simulink model "power_hvdc"  (Simulink 6.0)
settings: Solver=FixedStepDiscrete  SolverMode=SingleTasking  StartTime=0.0  StopTime=0.8  RelTol=1e-4
undefined symbols (not defined in the file or in its folder): D1, Delta
libraries: powerlib x28, powerlib_extras x7
settings Model: Creator=patrice  LastModifiedBy=batserve  ExtModeTrigMode=oneshot  ExtModeArmWhenConnect=off  ExtModeAutoUpdateStatusClock=off
settings DataIOCC: LimitDataPoints=off  SaveOutput=off  TimeSaveName=t  SignalLoggingName=sigsOut
settings OptimizationCC: BlockReduction=off  BooleanDataType=off
settings DebuggingCC: CheckExecutionContextPreStartOutputMsg=on  CheckExecutionContextRuntimeOutputMsg=on  SolverPrmCheckMsg=none
settings HardwareCC: TargetUnknown=on
settings RTWCC: TemplateMakefile=grt_unix.tmf

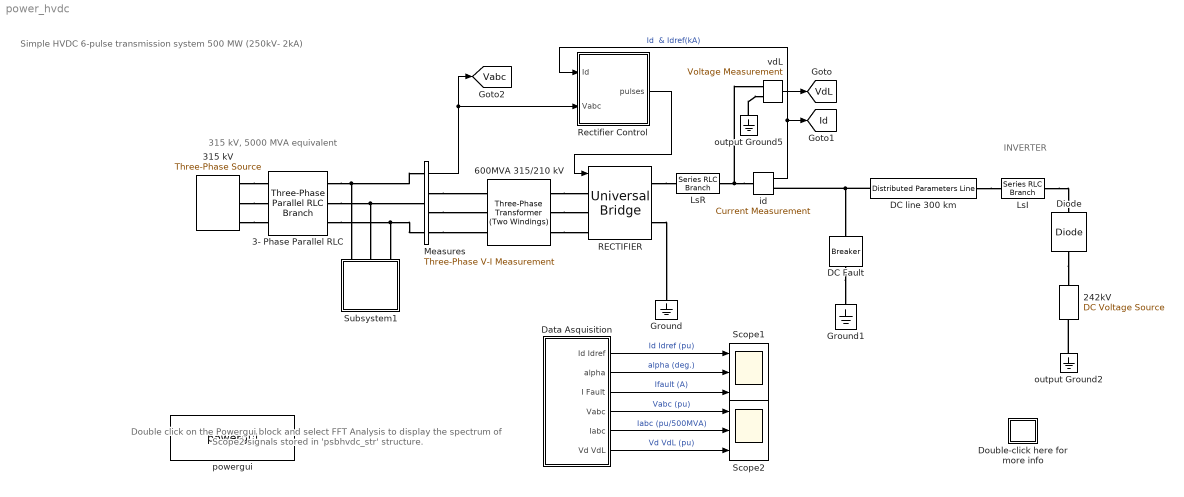
== system power_hvdc ==
  note: INVERTER
  note: Simple HVDC 6-pulse transmission system
      | 500 MW (250kV- 2kA)
  note: 315 kV, 5000 MVA equivalent
  note: Double click on the Powergui block
      | and select  FFT Analysis to display
      | the spectrum of Scope2  signals
      | stored in 'psbhvdc_str' structure.
  242kV : powerlib/Electrical Sources/DC Voltage Source  Description=source block  Orientation=up  Amplitude=242000  Measurements=None
      settings: AttributesFormatString=\n
  3- Phase Parallel RLC : powerlib/Elements/Three-Phase Parallel RLC Branch  PhysicalDomain=powersysdomain  SubClassName=unknown  LeftPortType=p1  RightPortType=p1  LConnTagsString=A|B|C  RConnTagsString=A|B|C  Resistance=12.41  Inductance=23.264e-3  Capacitance=0  Measurements=None
  315 kV : powerlib/Electrical Sources/Three-Phase Source  Voltage=315e3  PhaseAngle=0  Frequency=60  InternalConnection=Yg  SpecifyImpedance=off  Resistance=0  Inductance=46.671e-3  ShortCircuitLevel=0  BaseVoltage=0  XRratio=0
  600MVA 315/210 kV : powerlib/Elements/Three-Phase Transformer (Two Windings)  NominalPower=[ 600e6 60 ]  Winding1Connection=Yg  Winding1="[ 315e3*0.97 0.0015  0.0 ]"  Winding2Connection=Delta (D1)  Winding2=[ 210e3 0.0015 0.12]  SetSaturation=off  Rm=500  Lm=500  Saturation="[ 0,0  ;  0.005,1.2  ;  1.0,1.4 ]"  Hysteresis=off  DataFile='hysteresis'  SetInitialFlux=off  InitialFluxes=[ 0.8 , -0.8 , 0.7 ]  Measurements=None  TransfoNumber=0
  DC Fault : powerlib/Elements/Breaker  Orientation=down  BreakerResistance=0.1  InitialState=0  SnubberResistance=inf  SnubberCapacitance=0  SwitchingTimes=[ 0.5 0.51 ]  External=off  Measurements=Branch current
      settings: AttributesFormatString=\n
  DC line 300 km : powerlib/Elements/Distributed Parameters Line  Phases=1  Frequency=60  Resistance=0.015  Inductance=0.792e-3  Capacitance=14.4e-9  Length=300  x1=[0 0 0 0; 0.0001244 0 0 0; 0.0002488 0 0 0; 0.0003733 0 0 0; 0.0004977 0 0 0; 0.0006221 0 0 0]  x2=[0 0 0 0; 0.0001244 0 0 0; 0.0002488 0 0 0; 0.0003733 0 0 0; 0.0004977 0 0 0; 0.0006221 0 0 0]  x3=[0 0 0 0; 0.0001244 0 0 0; 0.0002488 0 0 0; 0.0003733 0 0 0; 0.0004977 0 0 0; 0.0006221 0 0 0]  x4=[0 0 0 0; 0.0001244 0 0 0; 0.0002488 0 0 0; 0.0003733 0 0 0; 0.0004977 0 0 0; 0.0006221 0 0 0]  x5=0  Measurements=None
      settings: AttributesFormatString=\n
  Data Asquisition : Subsystem
  Diode : powerlib/Power Electronics/Diode  Orientation=down  Ron=0.01  Lon=0  Vf=0.8  IC=0  Rs=1000  Cs=0.05e-6  Measurements=off
  Double-click here for more info : Subsystem
      mask Display: disp('?')
  Ground : powerlib/Elements/Ground  Orientation=down  PhysicalDomain=powersysdomain  SubClassName=unknown  LeftPortType=p1  RightPortType=p1  LConnTagsString=a
  Ground1 : powerlib/Elements/Ground  Orientation=down  PhysicalDomain=powersysdomain  SubClassName=unknown  LeftPortType=p1  RightPortType=p1  LConnTagsString=a
  LsI : powerlib/Elements/Series RLC Branch  PhysicalDomain=powersysdomain  SubClassName=unknown  LeftPortType=p1  RightPortType=p1  LConnTagsString=__new0  RConnTagsString=__new0  Resistance=.5  Inductance=.5  Capacitance=inf  Measurements=None
  "LsR " : powerlib/Elements/Series RLC Branch  PhysicalDomain=powersysdomain  SubClassName=unknown  LeftPortType=p1  RightPortType=p1  LConnTagsString=__new0  RConnTagsString=__new0  Resistance=.5  Inductance=.5  Capacitance=inf  Measurements=None
  Measures : powerlib/Measurements/Three-Phase V-I Measurement  VoltageMeasurement=phase-to-ground  SetLabelV=off  LabelV=V1  Vpu=on  Vbase=315e3  CurrentMeasurement=yes  SetLabelI=on  LabelI=Iabc  Ipu=on  Pbase=500e6  OutputType=Magnitude  PhasorSimulation=off  PSBequivalent=0
  RECTIFIER : powerlib/Power Electronics/Universal Bridge  Arms=3  SnubberResistance=2000  SnubberCapacitance=50e-9  Device=Thyristors  Ron=1e-3  Lon=0  ForwardVoltages="[  0.8  0.8  ]"  ForwardVoltage=0  GTOparameters=[ 10e-6 , 20e-6 ]  IGBTparameters=[ 1e-6 , 2e-6 ]  Measurements=UAB UBC UCA UDC voltages
  Rectifier Control : Subsystem
  Scope1 : Scope  NumInputPorts=3
      settings: TimeRange=0.8  YMin=-0.25~0~-500  YMax=2~170~6000  DataFormat=Array
  Scope2 : Scope  NumInputPorts=3
      settings: TimeRange=0.8  YMin=-1.5~-3~-1.5  YMax=1.5~3~2  SaveName=psbhvdc_str
  Subsystem1 : Subsystem  Orientation=down
      mask Display: disp('AC filters \n(320 Mvar)')
  id : powerlib/Measurements/Current Measurement  Tag=PoWeRsYsTeMmEaSuReMeNt  PhasorSimulation=off  OutputType=Complex  PSBequivalent=0
  output Ground2 : powerlib/Elements/Ground  Orientation=down  PhysicalDomain=powersysdomain  SubClassName=unknown  LeftPortType=p1  RightPortType=p1  LConnTagsString=a
  output Ground5 : powerlib/Elements/Ground  Orientation=down  PhysicalDomain=powersysdomain  SubClassName=unknown  LeftPortType=p1  RightPortType=p1  LConnTagsString=a
  powergui : powerlib/powergui  Priority=2  Frange=[0:2:500]  Ylog=off  Xlog=off  save=off  variable=ZData  structure=psbhvdc_str  ZoomFFT=on  StartTime=0.8-2/60  cycles=2  DisplayStyle=off  fundamental=60  FreqAxis=on  MaxFrequency=2000  frequencyindice=1  frequencyindicesteady=1  RmsSteady=1  display=off  Ts=1/360/64  methode=off  frequency=60  echomessages=off
  vdL : powerlib/Measurements/Voltage Measurement  Tag=PoWeRsYsTeMmEaSuReMeNt  PhasorSimulation=off  OutputType=Complex  PSBequivalent=0
  tag scope: Id=global, Vabc=global, VdL=global
  wires:
  Data Asquisition/6(Vd VdL) -> Scope2/3  "Vd VdL (pu)"
  Data Asquisition/1("Id Idref ") -> Scope1/1  "Id Idref (pu)"
  Data Asquisition/3(I Fault) -> Scope1/3  "Ifault (A)"
  Data Asquisition/2(alpha) -> Scope1/2  "alpha (deg.)"
  Data Asquisition/4(Vabc) -> Scope2/1  "Vabc (pu)"
  Data Asquisition/5(Iabc) -> Scope2/2  "Iabc (pu/500MVA)"
  Rectifier Control/1(pulses) -> RECTIFIER/1
  id/1 -> Rectifier Control/1(Id), [Id]  "Id  & Idref(kA)"
  Measures/1 -> [Vabc], Rectifier Control/2(Vabc)
  vdL/1 -> [VdL]
  connections:
  RECTIFIER/RConn1 -- "LsR "/LConn1
  RECTIFIER/RConn2 -- Ground/LConn1
  600MVA 315/210 kV/RConn1 -- RECTIFIER/LConn1
  600MVA 315/210 kV/RConn2 -- RECTIFIER/LConn2
  600MVA 315/210 kV/RConn3 -- RECTIFIER/LConn3
  Measures/RConn1 -- 600MVA 315/210 kV/LConn1
  Measures/RConn2 -- 600MVA 315/210 kV/LConn2
  Measures/RConn3 -- 600MVA 315/210 kV/LConn3
  DC line 300 km/RConn1 -- LsI/LConn1
  DC line 300 km/LConn1 -- id/RConn1 -- DC Fault/LConn1
  "LsR "/RConn1 -- id/LConn1 -- vdL/LConn1
  output Ground5/LConn1 -- vdL/LConn2
  DC Fault/RConn1 -- Ground1/LConn1
  output Ground2/LConn1 -- 242kV/LConn1
  LsI/RConn1 -- Diode/LConn1
  315 kV/RConn1 -- 3- Phase Parallel RLC/LConn1
  315 kV/RConn2 -- 3- Phase Parallel RLC/LConn2
  315 kV/RConn3 -- 3- Phase Parallel RLC/LConn3
  Diode/RConn1 -- 242kV/RConn1
  3- Phase Parallel RLC/RConn2 -- Measures/LConn2 -- Subsystem1/LConn2
  3- Phase Parallel RLC/RConn1 -- Measures/LConn1 -- Subsystem1/LConn1
  3- Phase Parallel RLC/RConn3 -- Measures/LConn3 -- Subsystem1/LConn3

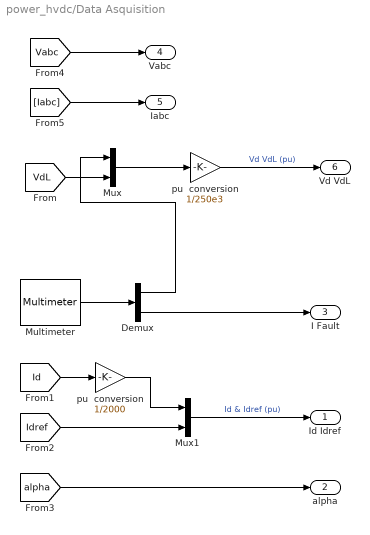
== system power_hvdc/Data Asquisition ==
  Demux : Demux  Outputs=2
  Multimeter : powerlib/Measurements/Multimeter  Tag=PoWeRsYsTeMmEaSuReMeNt  PhasorSimulation=off  OutputType=Magnitude  sel=[4 5]  L=5  Gain=[1 1]  yselected={'Udc: RECTIFIER','Ib: DC Fault'};  PSBOutputType=1  PSBequivalent=0  AxesSetting=[0,0.1,-100,100]  Display=0  SavedBlockNames={}
      settings: AttributesFormatString=\n
  Mux : Mux  Inputs=2
  Mux1 : Mux  Inputs=2
  pu  conversion : Gain  Gain=1/2000  SaturateOnIntegerOverflow=on
  "pu  conversion " : Gain  Gain=1/250e3  SaturateOnIntegerOverflow=on
  "Id Idref " : Outport
  alpha : Outport  Port=2
  I Fault : Outport  Port=3
  Vabc : Outport  Port=4
  Iabc : Outport  Port=5
  Vd VdL : Outport  Port=6
  wires:
  Mux/1 -> "pu  conversion "/1
  [VdL] -> Mux/2
  [Id] -> pu  conversion/1
  Mux1/1 -> "Id Idref "/1  "Id & Idref (pu)"
  [Idref] -> Mux1/2
  Demux/2 -> I Fault/1
  Demux/1 -> Mux/1
  [alpha] -> alpha/1
  [Vabc] -> Vabc/1
  [Iabc] -> Iabc/1
  "pu  conversion "/1 -> Vd VdL/1  "Vd VdL (pu)"
  pu  conversion/1 -> Mux1/1
  Multimeter/1 -> Demux/1

== system power_hvdc/Double-click here for more info ==
  note: Note: In oder to appreciate the speed improvemnt obtained with discretisation, you may try continuous simulation mode after completing this demo.
      |          The discrete system is approximately 6 times faster.
  note: Notice that the system is discretized (sample time 1/360/64 = 43.4 us). Setting, the sample time in to zero, will change to continuous integration for the power system .
  note: Frequency analysis of AC and DC voltages and currents
  note: In order to alllow further signal processing, signals displayed on Scope2 have been saved in a variable named 'psbvdc_str' ( structure with time').
      | These signals are : AC voltages (input 1) , AC currents (input 2) and DC voltages on rectifier and line side of the smoothing reactor (input 3).
      |
      | Open the Powergui and select  'FFT Analysis'. In the FFT window select structure 'psbhvdc_str'. The 0 - 2000 Hz FFT will be performed on  a 2-cycle window starting
      | at t = 0.8 - 2/60 (last 2 cycles of recording). Select input  labeled 'Iabc' . By default Phase a current (signal number 1) is selected. Press on 'Display' and observe
      |  the frequency spectrum of AC current. Harmonic currents (order 6n+/-1 , n = 1,2,3, ...for a 6-pulse converter) are displayed in % of the fundamental component .
      | If you analyze AC voltage (input Vabc) you shoud notice that the highest harmonics generated by the converter (5th and 7th) are filtered out by the two filters tuned at
      | the 5th and 7th harmonics.  Finally, select input labeled 'Vd VdL (pu)' and then input 1 or input 2.  You will obtain harmonic content (order 6n) of  the DC voltage Vd
      | (rectifier side) or VdL (line side) expressed in % of the DC component.
  note: G. Sybille (Hydro-Quebec)
  note: At t = 0.57 s, the regulator is released and it starts to regulate the DC current again. The steady-state 1 pu current is reached at t = 0.75 s.
  note: 0.57 < t < 0.8 s
  note: At t = 0.55 s, the alpha angle is forced by the protection system (not simulated) to reach 165 degrees when the Forced_alpha input of the current regulator goes high (1).
      | The rectifier thus passes in inverter mode and sends the energy stored in the line back to the 345 kV network.
      | As a result, the arc current producing the fault rapidly decreases . The fault is cleared at t = 0.555 s when the fault current zero crossing is reached.
  note: 0.55 < t <0.57 s
  note: At t = 0.5 s, a DC fault is applied on the line. The fault current ( trace 3) increases to 5 kA and the Id current increases to to 2 pu (4 kA) in 10 ms.
      | Then,  the fast regulator action lowers the current back to its reference value of 1 pu..
  note: 0.5 < t < 0.55 s
  note: 0.3 < t < 0.5 s
  note: At t = 0.3 s, the reference current is increased from  0.5 pu (1 kA) to the nominal current  1pu (2 kA). The current regulator  responds in approximately 0.1 s (6 cycles).
      | The alpha angle decreases from 30 degrees to 15 degrees.
  note: Trace 1 shows the the reference current (magenta) and the measured Id current (yellow). The reference current is set to 0.5 pu (1 kA). The DC current starts from zero
      | and reaches a steady-state in 0.1 s. Trace 2 shows the alpha firing angle required to obtain 0.5 pu of current (30 degrees).
  note: 0 < t < 0.3 s
  note: The system is programmed to start and  reach a steady state.  Then, a step is applied on the reference current to observe the dynamic response of the regulator.
      | Finally a DC fault is applied on the line.
      |
      | Start the simulation and observe the following events on  Scope1 :
  note: CIRCUIT DESCRIPTION
  note: This demonstration  illustrates steady-state and transient performance
      | of a simple 500 MW (250 kV-2kA) HVDC transmission system
  note: A 500 MW (250 kV, 2 kA) DC linterconnexion is used to transmit power from a 315 kV, 5000 MVA AC network. The network is simulated by a LLR damped equivalent
      | (impedance angle of 80 degrees at 60 Hz and 3rd harmonic). The converter transformer  and the rectifier are modelled respectively with the Universal Transformer
      | and Universal Bridge blocks The converter is a 6-pulse rectifier. It is connected to a 300 km distributed parameter line through a 0.5 H smoothing reactor LsR.
      | The inverter is simulated by a simple DC voltage source in series with a diode (to force unidirectional conduction) and smoothing reactor LsI.
      | The reactive power required by the converter is provided by a set of filters (C bank plus 5th, 7th and high pass filters; total 320 Mvar).
      | Open the AC filter subsystem to see the filter toplogy.  A circuit breaker allows to apply a DC line fault on the rectifier side.
      |
      | The control system uses two main blocks: the Synchronized 6-pulse generator of the Extras/Control library and a PI Curent Regulator.
      | Voltages sent to the synchronization system are filtered by 2nd order band pass filters. The whole control system is discretized (Sample time = 1/360/64 = 43.4 us).
      |
      | THe DC line current at the output of the rectifier is compared with a reference. The PI regulator tries to keep the error at zero and outputs the alpha firing angle required
      | by the synchronizing unit. Inputs 3 and 4 of the current regulator allow to bypass the regulator action and to impose the alpha firing angle
  note: DEMONSTRATION

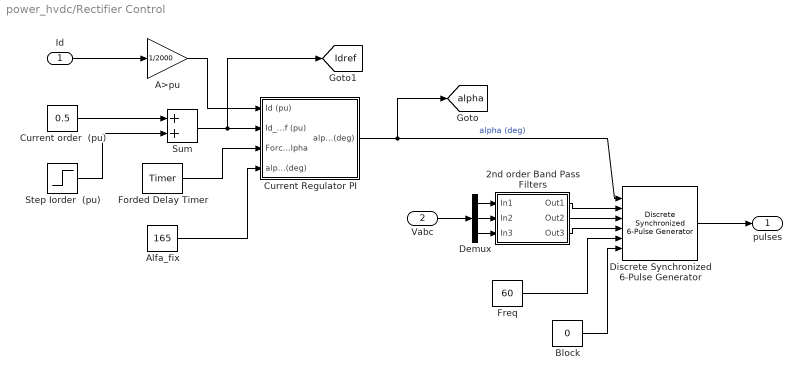
== system power_hvdc/Rectifier Control ==
  Id : Inport  Port=1  LatchInput=off
  Vabc : Inport  Port=2  LatchInput=off
  2nd order Band Pass Filters : Subsystem
      mask Display:
      | disp(' Fo=60 Hz\n\n
      | BW=30 Hz')
  A>pu : Gain  Gain=1/2000  SaturateOnIntegerOverflow=on
  Alfa_fix : Constant  Value=165
  Block : Constant  Value=0
  Current Regulator PI : Subsystem
  Current order  (pu) : Constant  Value=0.5
  Demux : Demux  Outputs=3
  Discrete Synchronized 6-Pulse Generator : powerlib_extras/Discrete  Control Blocks/Discrete Synchronized 6-Pulse Generator  pwidth=70  Double_Pulse=off  Ts=1/360/64
  Forded Delay Timer : powerlib_extras/Control  Blocks/Timer  t=[ 0.55 0.57]  e="[1 0  ]"
  Freq : Constant  Value=60
  "Step Iorder  (pu)  " : Step  Time=0.3  After=0.6  SampleTime=0  ZeroCross=off
  Sum : Sum  SaturateOnIntegerOverflow=on  InputSameDT=on
  pulses : Outport
  tag scope: Idref=global, alpha=global
  wires:
  Demux/1 -> 2nd order Band Pass Filters/1(In1)
  Demux/3 -> 2nd order Band Pass Filters/3(In3)
  Demux/2 -> 2nd order Band Pass Filters/2(In2)
  2nd order Band Pass Filters/2(Out2) -> Discrete Synchronized 6-Pulse Generator/3
  2nd order Band Pass Filters/1(Out1) -> Discrete Synchronized 6-Pulse Generator/2
  2nd order Band Pass Filters/3(Out3) -> Discrete Synchronized 6-Pulse Generator/4
  Block/1 -> Discrete Synchronized 6-Pulse Generator/6
  Freq/1 -> Discrete Synchronized 6-Pulse Generator/5
  Vabc/1 -> Demux/1
  Discrete Synchronized 6-Pulse Generator/1 -> pulses/1
  Current order  (pu)/1 -> Sum/1
  "Step Iorder  (pu)  "/1 -> Sum/2
  Sum/1 -> Current Regulator PI/2(Id_ref (pu)), [Idref]
  A>pu/1 -> Current Regulator PI/1(Id (pu))
  Current Regulator PI/1(alpha (deg)) -> Discrete Synchronized 6-Pulse Generator/1, [alpha]  "alpha (deg)"
  Alfa_fix/1 -> Current Regulator PI/4(alpha_fix(deg))
  Forded Delay Timer/1 -> Current Regulator PI/3(Forced_alpha)
  Id/1 -> A>pu/1

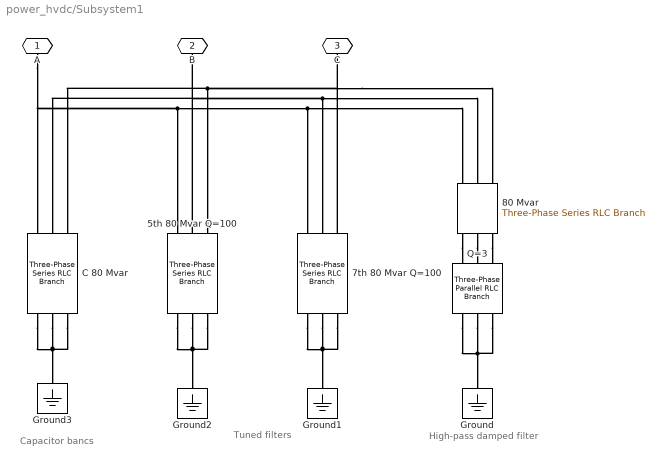
== system power_hvdc/Subsystem1 ==
  note: High-pass
      | damped filter
  note: Tuned filters
  note: Capacitor bancs
  "5th 80 Mvar Q=100 " : powerlib/Elements/Three-Phase Series RLC Branch  Orientation=down  PhysicalDomain=powersysdomain  SubClassName=unknown  LeftPortType=p1  RightPortType=p1  LConnTagsString=A|B|C  RConnTagsString=A|B|C  Resistance=2.48  Inductance=131.5e-3  Capacitance=2.14e-6  Measurements=None
  7th 80 Mvar Q=100 : powerlib/Elements/Three-Phase Series RLC Branch  Orientation=down  PhysicalDomain=powersysdomain  SubClassName=unknown  LeftPortType=p1  RightPortType=p1  LConnTagsString=A|B|C  RConnTagsString=A|B|C  Resistance=1.77  Inductance=67.1e-3  Capacitance=2.14e-6  Measurements=None
  80 Mvar : powerlib/Elements/Three-Phase Series RLC Branch  Orientation=down  PhysicalDomain=powersysdomain  SubClassName=unknown  LeftPortType=p1  RightPortType=p1  LConnTagsString=A|B|C  RConnTagsString=A|B|C  Resistance=0  Inductance=0  Capacitance=2.14e-6  Measurements=None
  C 80 Mvar : powerlib/Elements/Three-Phase Series RLC Branch  Orientation=down  PhysicalDomain=powersysdomain  SubClassName=unknown  LeftPortType=p1  RightPortType=p1  LConnTagsString=A|B|C  RConnTagsString=A|B|C  Resistance=0  Inductance=0  Capacitance=2.14e-6  Measurements=None
  Ground{,1..3} (4 alike) : powerlib/Elements/Ground  Orientation=down  PhysicalDomain=powersysdomain  SubClassName=unknown  LeftPortType=p1  RightPortType=p1  LConnTagsString=a
  Q=3 : powerlib/Elements/Three-Phase Parallel RLC Branch  Orientation=down  PhysicalDomain=powersysdomain  SubClassName=unknown  LeftPortType=p1  RightPortType=p1  LConnTagsString=A|B|C  RConnTagsString=A|B|C  Resistance=225.6  Inductance=27.2e-3  Capacitance=0  Measurements=None
  A : PMIOPort  Orientation=down  Port=1  Side=Left
  B : PMIOPort  Orientation=down  Port=2  Side=Left
  C : PMIOPort  Orientation=down  Port=3  Side=Left
  connections:
  80 Mvar/RConn3 -- Q=3/LConn3
  80 Mvar/RConn2 -- Q=3/LConn2
  80 Mvar/RConn1 -- Q=3/LConn1
  "5th 80 Mvar Q=100 "/RConn3 -- "5th 80 Mvar Q=100 "/RConn2 -- Ground2/LConn1 -- "5th 80 Mvar Q=100 "/RConn1
  C 80 Mvar/RConn3 -- C 80 Mvar/RConn2 -- Ground3/LConn1 -- C 80 Mvar/RConn1
  Q=3/RConn2 -- Ground/LConn1 -- Q=3/RConn3 -- Q=3/RConn1
  7th 80 Mvar Q=100/RConn3 -- 7th 80 Mvar Q=100/RConn2 -- Ground1/LConn1 -- 7th 80 Mvar Q=100/RConn1
  A/RConn1 -- C 80 Mvar/LConn1 -- 80 Mvar/LConn1 -- 7th 80 Mvar Q=100/LConn1 -- "5th 80 Mvar Q=100 "/LConn1
  "5th 80 Mvar Q=100 "/LConn2 -- B/RConn1 -- C 80 Mvar/LConn2 -- 80 Mvar/LConn2 -- 7th 80 Mvar Q=100/LConn2
  7th 80 Mvar Q=100/LConn3 -- C/RConn1 -- 80 Mvar/LConn3 -- C 80 Mvar/LConn3 -- "5th 80 Mvar Q=100 "/LConn3

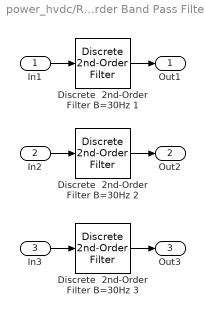
== system power_hvdc/Rectifier Control/2nd order Band Pass Filters ==
  In1 : Inport  Port=1  LatchInput=off
  In2 : Inport  Port=2  LatchInput=off
  In3 : Inport  Port=3  LatchInput=off
  Discrete  2nd-Order Filter B=30Hz 1 : powerlib_extras/Discrete  Control Blocks/Discrete  2nd-Order Filter  FilterType=Bandpass  Fo=60  Zeta=0.25  Ts=1/360/64  Initialize=on  Vac_Init=[0.8 -25 60]  Vdc_Init=-0.4  PlotResponse=off  param1=[1 500 0.1]
  Discrete  2nd-Order Filter B=30Hz 2 : powerlib_extras/Discrete  Control Blocks/Discrete  2nd-Order Filter  FilterType=Bandpass  Fo=60  Zeta=0.25  Ts=1/360/64  Initialize=on  Vac_Init=[0.8 -25 60]  Vdc_Init=-0.4  PlotResponse=off  param1=[1 500 0.1]
  Discrete  2nd-Order Filter B=30Hz 3 : powerlib_extras/Discrete  Control Blocks/Discrete  2nd-Order Filter  FilterType=Bandpass  Fo=60  Zeta=0.25  Ts=1/360/64  Initialize=on  Vac_Init=[0.8 -25 60]  Vdc_Init=-0.4  PlotResponse=off  param1=[1 500 0.1]
  Out1 : Outport
  Out2 : Outport  Port=2
  Out3 : Outport  Port=3
  wires:
  Discrete  2nd-Order Filter B=30Hz 1/1 -> Out1/1
  In1/1 -> Discrete  2nd-Order Filter B=30Hz 1/1
  In2/1 -> Discrete  2nd-Order Filter B=30Hz 2/1
  In3/1 -> Discrete  2nd-Order Filter B=30Hz 3/1
  Discrete  2nd-Order Filter B=30Hz 2/1 -> Out2/1
  Discrete  2nd-Order Filter B=30Hz 3/1 -> Out3/1

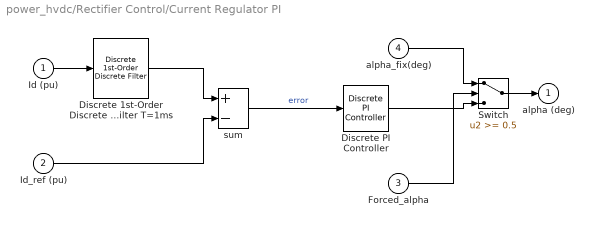
== system power_hvdc/Rectifier Control/Current Regulator PI ==
  Id (pu) : Inport  Port=1  LatchInput=off
  Id_ref (pu) : Inport  Port=2  LatchInput=off
  Forced_alpha : Inport  Port=3  LatchInput=off
  alpha_fix(deg) : Inport  Port=4  LatchInput=off
  Discrete 1st-Order Discrete Filter T=1ms : powerlib_extras/Discrete  Control Blocks/Discrete 1st-Order Discrete Filter  FilterType=Lowpass  Tc=1e-3  Ts=1/360/64  Initialize=off  Vac_Init=[0.8 -25 60]  Vdc_Init=-0.4  PlotResponse=off  param1=[1 500 0.1]
  Discrete PI Controller : powerlib_extras/Discrete  Control Blocks/Discrete PI Controller  Kp=65  Ki=5000  Par_Limits=[165 5]  Init=90  Ts=1/360/64
  Switch : Switch  Threshold=0.5  ZeroCross=off  InputSameDT=on
  sum : Sum  Inputs=+-  SaturateOnIntegerOverflow=on  InputSameDT=on
  alpha (deg) : Outport  InitialOutput=0
  wires:
  Id_ref (pu)/1 -> sum/2
  Discrete 1st-Order Discrete Filter T=1ms/1 -> sum/1
  Id (pu)/1 -> Discrete 1st-Order Discrete Filter T=1ms/1
  sum/1 -> Discrete PI Controller/1  "error"
  Forced_alpha/1 -> Switch/2
  Switch/1 -> alpha (deg)/1
  alpha_fix(deg)/1 -> Switch/1
  Discrete PI Controller/1 -> Switch/3
